simulink model "DCservo"  (R2016a)
settings: Solver=VariableStepAuto  StartTime=0.0  StopTime=10.0  MaxStep=.01  RelTol=1e-3
settings Model: Creator=jordan  LastModifiedBy=jordan
settings DataIOCC: SaveOutput=off  SaveTime=off

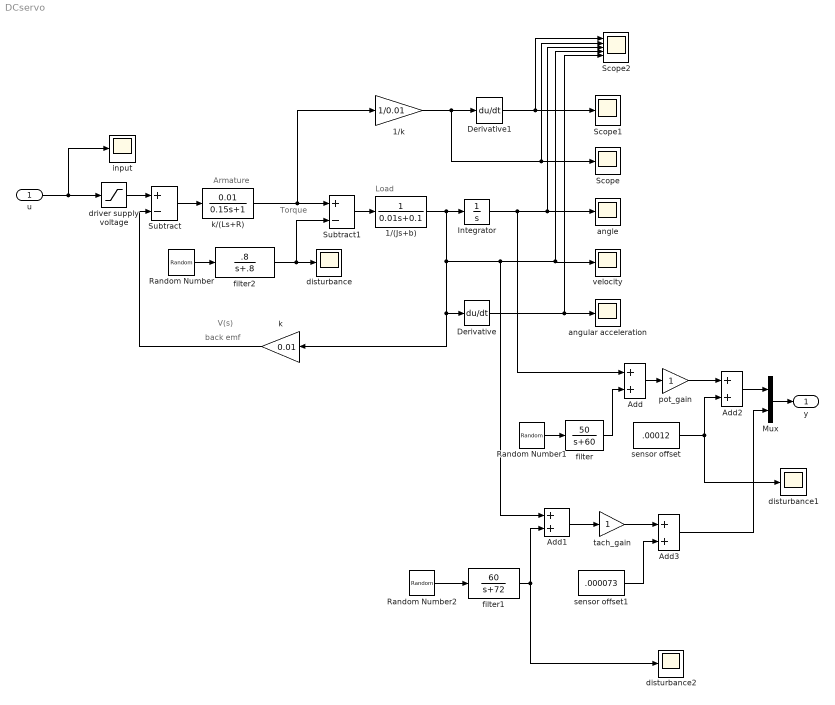
== system DCservo ==
  note: back emf
  note: Armature
  note: Torque
  note: Load
  note: V(s)
  u : Inport  OutDataTypeStr=double  PortDimensions=1  SampleTime=0
  1/(Js+b) : TransferFcn  Denominator=[0.01 0.1]
  1/k : Gain  Gain=1/0.01
  Add{,1..3} (4 alike) : Sum
  Derivative : Derivative
  Derivative1 : Derivative
  Integrator : Integrator
  Mux : Mux  Inputs=2
  Random Number : RandomNumber  Variance=.0000018
  Random Number1 : RandomNumber  Variance=.0000011
  Random Number2 : RandomNumber  Variance=.0000017
  Scope : Scope
  Scope1 : Scope
  Scope2 : Scope  NumInputPorts=5
  Subtract : Sum  Inputs=+-
  Subtract1 : Sum  Inputs=+-
  angle : Scope
  angular acceleration : Scope
  disturbance : Scope
  disturbance1 : Scope
  disturbance2 : Scope
  driver supply voltage : Saturate  UpperLimit=12  LowerLimit=-12
  filter : TransferFcn  Numerator=[50]  Denominator=[1 60]
  filter1 : TransferFcn  Numerator=[60]  Denominator=[1 72]
  filter2 : TransferFcn  Numerator=[.8]  Denominator=[1 .8]
  input : Scope
  k : Gain  Gain=0.01
  k/(Ls+R) : TransferFcn  Numerator=[0.01]  Denominator=[0.15 1]
  pot_gain : Gain
  sensor offset : Constant  Value=.00012
  sensor offset1 : Constant  Value=.000073
  tach_gain : Gain
  velocity : Scope
  y : Outport  OutDataTypeStr=double  PortDimensions=2  SampleTime=0
  wires:
  k/(Ls+R)/1 -> Subtract1/1, 1/k/1
  1/(Js+b)/1 -> k/1, Derivative/1, Add1/1, Scope2/4, velocity/1, Integrator/1
  Integrator/1 -> Add/1, Scope2/3, angle/1
  k/1 -> Subtract/2
  Subtract/1 -> k/(Ls+R)/1
  Derivative/1 -> Scope2/5, angular acceleration/1
  1/k/1 -> Derivative1/1, Scope/1, Scope2/2
  Derivative1/1 -> Scope2/1, Scope1/1
  Mux/1 -> y/1
  driver supply voltage/1 -> Subtract/1
  Add/1 -> pot_gain/1
  Add1/1 -> tach_gain/1
  Random Number1/1 -> filter/1
  Random Number2/1 -> filter1/1
  filter/1 -> Add/2
  filter1/1 -> disturbance2/1, Add1/2
  pot_gain/1 -> Add2/1
  Add2/1 -> Mux/1
  tach_gain/1 -> Add3/1
  Add3/1 -> Mux/2
  sensor offset/1 -> Add2/2, disturbance1/1
  sensor offset1/1 -> Add3/2
  u/1 -> driver supply voltage/1, input/1
  Random Number/1 -> filter2/1
  filter2/1 -> Subtract1/2, disturbance/1
  Subtract1/1 -> 1/(Js+b)/1
